simulink model "sim_exp_sim"  (Simulink 8.9)
settings: Solver=ode23s  StartTime=0.0  StopTime=T_sweep  RelTol=1e-3
values from neighbouring files (symbols this model uses):
  dgr = 0.65    [main_sim_exp.m]
  dgs = 6    [main_sim_exp.m]
  f_log = 1000    [main_sim_exp.m]
  Jl = 1.2 * Jl    (= 0.0491496)    [main_sim_exp.m]
  Jsint = scale*Jsint    (= 0.00011)    [main_sim_exp.m]
  Jtot = [0.000306 +  0.28200e-04]    [main_sim_exp.m]
  kg = 2.7e4    (= 27000)    [main_sim_exp.m]
  ks = 8.1853e4*1.4    (= 114594.2)    [main_sim_exp.m]
  rg = 160    [main_sim_exp.m]
  Vel_mot_nom = 263    [main_sim_exp.m]
libraries: simulink x1
settings Model: Creator=eshojaei  LastModifiedBy=Gustavo
settings DataIOCC: LimitDataPoints=off  SaveFormat=Dataset  SignalLoggingSaveFormat=Dataset
settings OptimizationCC: LifeSpan=auto
settings DebuggingCC: UnderspecifiedInitializationDetection=Simplified  MergeDetectMultiDrivingBlocksExec=error  FcnCallInpInsideContextMsg=error  StateNameClashWarn=none  SFUnexpectedBacktrackingDiag=error  SFNoUnconditionalDefaultTransitionDiag=error  SFExecutionAtInitializationDiag=warning
settings HardwareCC: ProdBitPerPointer=64  ProdBitPerSizeT=64  ProdBitPerPtrDiffT=64  ProdLargestAtomicFloat=Float  ProdIntDivRoundTo=Zero  ProdEndianess=LittleEndian  ProdWordSize=64  ProdHWDeviceType=Intel->x86-64 (Windows64)
settings ModelReferenceCC: PropagateSignalLabelsOutOfModel=on
settings SFSimCC: SimUseLocalCustomCode=on
settings RTWCC: RTWUseLocalCustomCode=on
settings GRTTargetCC: TargetLangStandard=C99 (ISO)  GeneratePreprocessorConditionals=Use local settings  CombineOutputUpdateFcns=on  GRTInterface=off
settings ConfigComp: CovMetricSettings=dwe  CovHtmlReporting=off  CovSaveCumulativeToWorkspaceVar=off  CovSaveSingleToWorkspaceVar=off  CovExternalEMLEnable=on

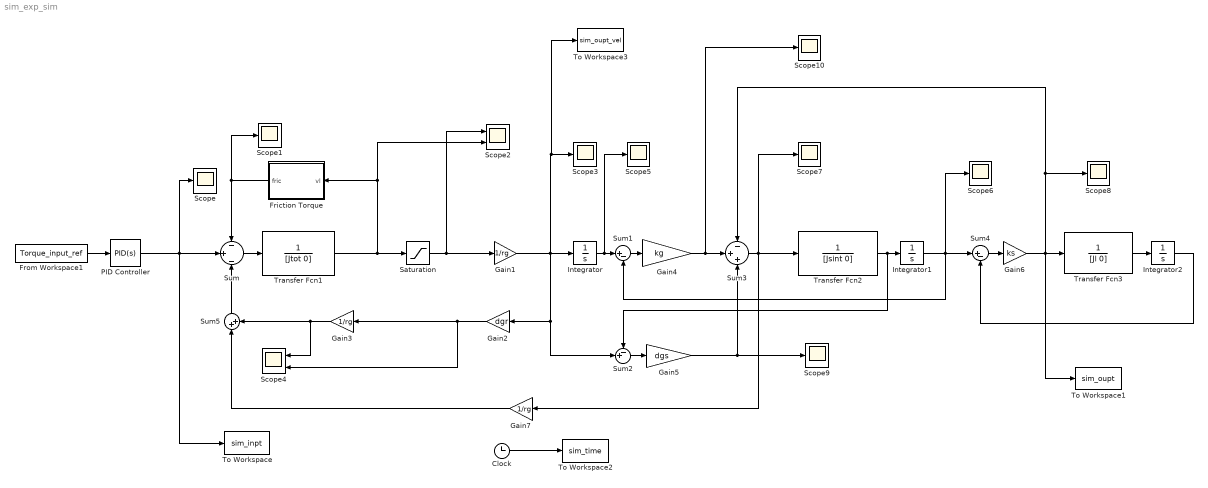
== system sim_exp_sim ==
  Clock : Clock
  Friction Torque : MATLAB Function  TreatAsAtomicUnit=on
  From Workspace1 : FromWorkspace  VariableName=Torque_input_ref  SampleTime=0.001
  Gain1 : Gain  Gain=1/rg
  Gain2 : Gain  Gain=dgr
  Gain3 : Gain  Gain=1/rg
  Gain4 : Gain  Gain=kg
  Gain5 : Gain  Gain=dgs
  Gain6 : Gain  Gain=ks
  Gain7 : Gain  Gain=1/rg
  Integrator : Integrator
  Integrator1 : Integrator
  Integrator2 : Integrator
  PID Controller : simulink/Continuous/PID Controller  Controller=PID  TimeDomain=Continuous-time  SampleTime=-1  IntegratorMethod=Forward Euler  FilterMethod=Forward Euler  Form=Parallel  UseFilter=on  ControllerParametersSource=internal  P=1  I=0  D=0  N=100  InitialConditionSource=internal  InitialConditionForIntegrator=0  InitialConditionForFilter=0  ExternalReset=none  LimitOutput=off  UpperSaturationLimit=inf  LowerSaturationLimit=-inf  LinearizeAsGain=on  AntiWindupMode=none  Kb=1  TrackingMode=off  Kt=1  PParamMin=[]  PParamMax=[]  IParamMin=[]  IParamMax=[]  DParamMin=[]  DParamMax=[]  NParamMin=[]  NParamMax=[]  KbParamMin=[]  KbParamMax=[]  KtParamMin=[]  KtParamMax=[]  POutMin=[]  POutMax=[]  IOutMin=[]  IOutMax=[]  DOutMin=[]  DOutMax=[]  NOutMin=[]  NOutMax=[]  KbOutMin=[]  KbOutMax=[]  KtOutMin=[]  KtOutMax=[]  IntegratorOutMin=[]  IntegratorOutMax=[]  FilterOutMin=[]  FilterOutMax=[]  SumOutMin=[]  SumOutMax=[]  SumI1OutMin=[]  SumI1OutMax=[]  SumI2OutMin=[]  SumI2OutMax=[]  SumI3OutMin=[]  SumI3OutMax=[]  SumDOutMin=[]  SumDOutMax=[]  SaturationOutMin=[]  SaturationOutMax=[]  IntegratorContinuousStateAttributes=''  IntegratorStateMustResolveToSignalObject=off  IntegratorRTWStateStorageClass=Auto  FilterContinuousStateAttributes=''  FilterStateMustResolveToSignalObject=off  FilterRTWStateStorageClass=Auto  DifferentiatorICPrevScaledInput=0  DifferentiatorOutMin=[]  DifferentiatorOutMax=[]
  Saturation : Saturate  UpperLimit=Vel_mot_nom  LowerLimit=-Vel_mot_nom
  Scope{,1,3,5..10} (9 alike) : Scope
  Scope2 : Scope  NumInputPorts=2
  Scope4 : Scope  NumInputPorts=2
  Sum : Sum  Inputs=-|+|-
  Sum1 : Sum  Inputs=|+-
  Sum2 : Sum  Inputs=-+|
  Sum3 : Sum  Inputs=-++
  Sum4 : Sum  Inputs=|+-
  Sum5 : Sum  Inputs=|++
  To Workspace : ToWorkspace  VariableName=sim_inpt  SaveFormat=Timeseries  SampleTime=1/f_log
  To Workspace1 : ToWorkspace  VariableName=sim_oupt  SaveFormat=Timeseries  SampleTime=1/f_log
  To Workspace2 : ToWorkspace  VariableName=sim_time  SaveFormat=Timeseries  SampleTime=1/f_log
  To Workspace3 : ToWorkspace  VariableName=sim_oupt_vel  SaveFormat=Timeseries  SampleTime=1/f_log
  Transfer Fcn1 : TransferFcn  Denominator=[Jtot 0]
  Transfer Fcn2 : TransferFcn  Denominator=[Jsint 0]
  Transfer Fcn3 : TransferFcn  Denominator=[Jl 0]
  wires:
  PID Controller/1 -> Scope/1, To Workspace/1, Sum/2
  Transfer Fcn1/1 -> Saturation/1, Friction Torque/1(vl), Scope2/2
  Saturation/1 -> Gain1/1, Scope2/1
  Friction Torque/1(fric) -> Sum/1, Scope1/1
  Sum/1 -> Transfer Fcn1/1
  Gain1/1 -> To Workspace3/1, Scope3/1, Integrator/1, Sum2/2, Gain2/1
  Gain2/1 -> Scope4/2, Gain3/1
  Gain3/1 -> Sum5/2, Scope4/1
  Integrator/1 -> Sum1/1, Scope5/1
  Sum1/1 -> Gain4/1
  Transfer Fcn2/1 -> Sum2/1, Integrator1/1
  Integrator1/1 -> Sum4/1, Scope6/1, Sum1/2
  Sum2/1 -> Gain5/1
  Sum3/1 -> Gain7/1, Transfer Fcn2/1, Scope7/1
  Sum4/1 -> Gain6/1
  Transfer Fcn3/1 -> Integrator2/1
  Integrator2/1 -> Sum4/2
  Sum5/1 -> Sum/3
  Clock/1 -> To Workspace2/1
  Gain7/1 -> Sum5/1
  Gain4/1 -> Scope10/1, Sum3/2
  Gain5/1 -> Sum3/3, Scope9/1
  Gain6/1 -> To Workspace1/1, Sum3/1, Scope8/1, Transfer Fcn3/1
  From Workspace1/1 -> PID Controller/1

== matlab function Friction Torque ==
  data: vl input double; fric output double
function fric = fcn(vl)

    
   fric = (5981672325465929*vl)/147573952589676412928 + (7059617857129123*tanh((6072588977179245*vl)/36028797018963968))/144115188075855872 + (2558104915892175*tanh((5176012883402097*vl)/576460752303423488))/72057594037927936;
